simulink model "Moteur"  (Simulink 10.1)
settings: Solver=FixedStepAuto  StartTime=0.0  StopTime=5  FixedStep=1e-6  RelTol=1e-3  EnableMultiTasking=on
settings Model: Creator=SINA  LastModifiedBy=SINA
settings DataIOCC: SaveFormat=Dataset
settings DebuggingCC: UnderspecifiedInitializationDetection=Simplified  MergeDetectMultiDrivingBlocksExec=error  SFExecutionAtInitializationDiag=warning
settings HardwareCC: ProdBitPerPointer=64  ProdBitPerSizeT=64  ProdBitPerPtrDiffT=64  ProdLargestAtomicFloat=Float  ProdIntDivRoundTo=Zero  ProdEndianess=LittleEndian  ProdWordSize=64  ProdHWDeviceType=Intel->x86-64 (Windows64)
settings ModelReferenceCC: PropagateSignalLabelsOutOfModel=on
settings GRTTargetCC: CombineOutputUpdateFcns=on  GRTInterface=off
settings SimscapeCC: SimscapeNormalizeSystem=off

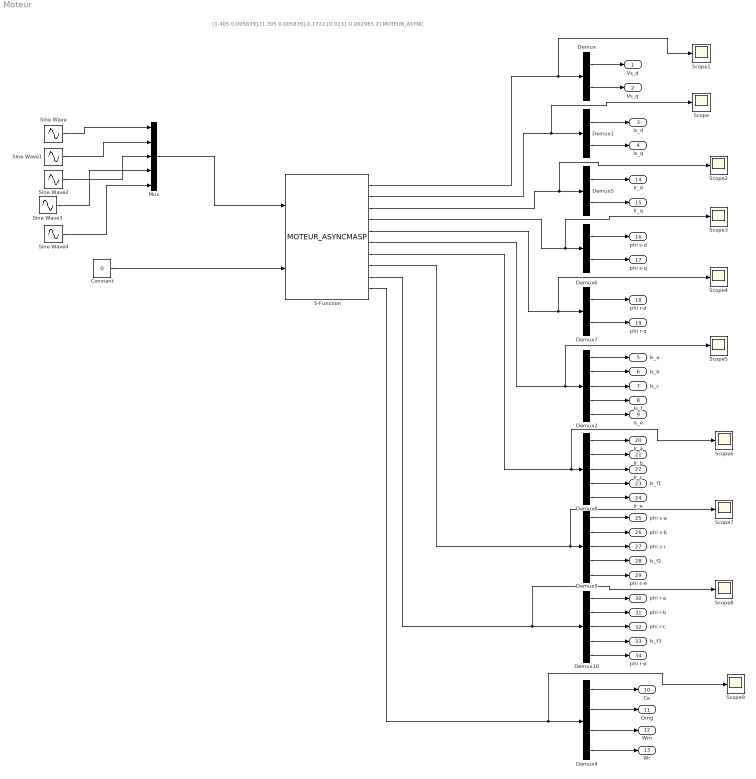
== system Moteur ==
  note: [1.405 0.005839],[1.395 0.005839],0.1722,[0.0131 0.002985 2]
      | MOTEUR_ASYNC
  Constant : Constant  Value=0
  Demux{,1,5..7} (5 alike) : Demux  Outputs=2
  Demux{2,8..10} (4 alike) : Demux  Outputs=5
  Demux4 : Demux
  Mux : Mux  Inputs=5
  S-Function : S-Function  FunctionName=MOTEUR_ASYNCMASP  Parameters=[1.405 0.005839],[1.395 0.005839],0.1722,[0.0131 0.002985 2]  SFunctionDeploymentMode=off  EnableBusSupport=off
  Scope{,1..9} (10 alike) : Scope
  Sine Wave : Sin  Amplitude=400  Frequency=2*pi*50  SampleTime=0
  Sine Wave1 : Sin  Amplitude=400  Frequency=2*pi*50  Phase=2*pi/5  SampleTime=0
  Sine Wave2 : Sin  Amplitude=400  Frequency=2*pi*50  Phase=4*pi/5  SampleTime=0
  Sine Wave3 : Sin  Amplitude=400  Frequency=2*pi*50  Phase=6*pi/5  SampleTime=0
  Sine Wave4 : Sin  Amplitude=400  Frequency=2*pi*50  Phase=8*pi/5  SampleTime=0
  Vs_d : Outport
  Vs_q : Outport  Port=2
  Is_d : Outport  Port=3
  Is_q : Outport  Port=4
  Is_a : Outport  Port=5
  Is_b : Outport  Port=6
  Is_c : Outport  Port=7
  Is_f : Outport  Port=8
  Is_e : Outport  Port=9
  Ce : Outport  Port=10
  Omg : Outport  Port=11
  Wm : Outport  Port=12
  Wr : Outport  Port=13
  Ir_d : Outport  Port=14
  Ir_q : Outport  Port=15
  phi s-d : Outport  Port=16
  phi s-q : Outport  Port=17
  phi r-d : Outport  Port=18
  phi r-q : Outport  Port=19
  Ir_a : Outport  Port=20
  Ir_b : Outport  Port=21
  Ir_c : Outport  Port=22
  Is_f1 : Outport  Port=23
  Ir_e : Outport  Port=24
  phi s-a : Outport  Port=25
  phi s-b : Outport  Port=26
  phi s-c : Outport  Port=27
  Is_f2 : Outport  Port=28
  phi s-e : Outport  Port=29
  phi r-a : Outport  Port=30
  phi r-b : Outport  Port=31
  phi r-c : Outport  Port=32
  Is_f3 : Outport  Port=33
  phi r-e : Outport  Port=34
  wires:
  Constant/1 -> S-Function/2
  Demux2/3 -> Is_c/1
  Demux2/2 -> Is_b/1
  Demux2/1 -> Is_a/1
  Demux1/2 -> Is_q/1
  Demux1/1 -> Is_d/1
  Demux/2 -> Vs_q/1
  Demux/1 -> Vs_d/1
  Sine Wave1/1 -> Mux/2
  Sine Wave2/1 -> Mux/3
  Mux/1 -> S-Function/1
  Sine Wave/1 -> Mux/1
  Demux2/4 -> Is_f/1
  Demux2/5 -> Is_e/1
  Sine Wave4/1 -> Mux/5
  Sine Wave3/1 -> Mux/4
  Demux5/1 -> Ir_d/1
  Demux5/2 -> Ir_q/1
  Demux6/1 -> phi s-d/1
  Demux7/1 -> phi r-d/1
  Demux7/2 -> phi r-q/1
  S-Function/1 -> Scope1/1, Demux/1
  S-Function/2 -> Scope/1, Demux1/1
  S-Function/3 -> Scope2/1, Demux5/1
  S-Function/5 -> Scope4/1, Demux7/1
  Demux6/2 -> phi s-q/1
  S-Function/4 -> Scope3/1, Demux6/1
  S-Function/6 -> Scope5/1, Demux2/1
  Demux8/5 -> Ir_e/1
  Demux8/4 -> Is_f1/1
  Demux8/1 -> Ir_a/1
  Demux8/2 -> Ir_b/1
  Demux8/3 -> Ir_c/1
  S-Function/7 -> Scope6/1, Demux8/1
  Demux9/3 -> phi s-c/1
  Demux9/2 -> phi s-b/1
  Demux9/1 -> phi s-a/1
  Demux9/4 -> Is_f2/1
  Demux9/5 -> phi s-e/1
  Demux10/5 -> phi r-e/1
  Demux10/4 -> Is_f3/1
  Demux10/1 -> phi r-a/1
  Demux10/2 -> phi r-b/1
  Demux10/3 -> phi r-c/1
  S-Function/8 -> Scope7/1, Demux9/1
  S-Function/9 -> Scope8/1, Demux10/1
  S-Function/10 -> Scope9/1, Demux4/1
  Demux4/1 -> Ce/1
  Demux4/2 -> Omg/1
  Demux4/3 -> Wm/1
  Demux4/4 -> Wr/1
